simulink model "FW_control"  (R2023b)
settings: Solver=ode45  StartTime=0.0  StopTime=100  RelTol=1e-3
libraries: Fixed_Wing x2
settings Model: Creator=TigerWuu  LastModifiedBy=NCS
settings DebuggingCC: UnconnectedInputMsg=warning  UnconnectedOutputMsg=warning  UnconnectedLineMsg=warning
settings ModelReferenceCC: EnableRefExpFcnMdlSchedulingChecks=on
settings RTWCC: DLArmComputeVersion=19.05

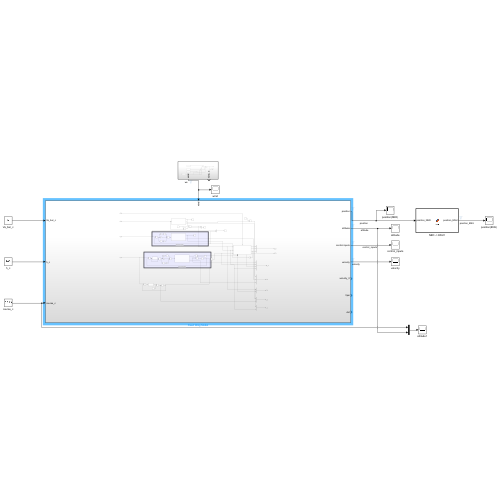
[thumbnail: Simulink's stored preview of the top-level diagram]
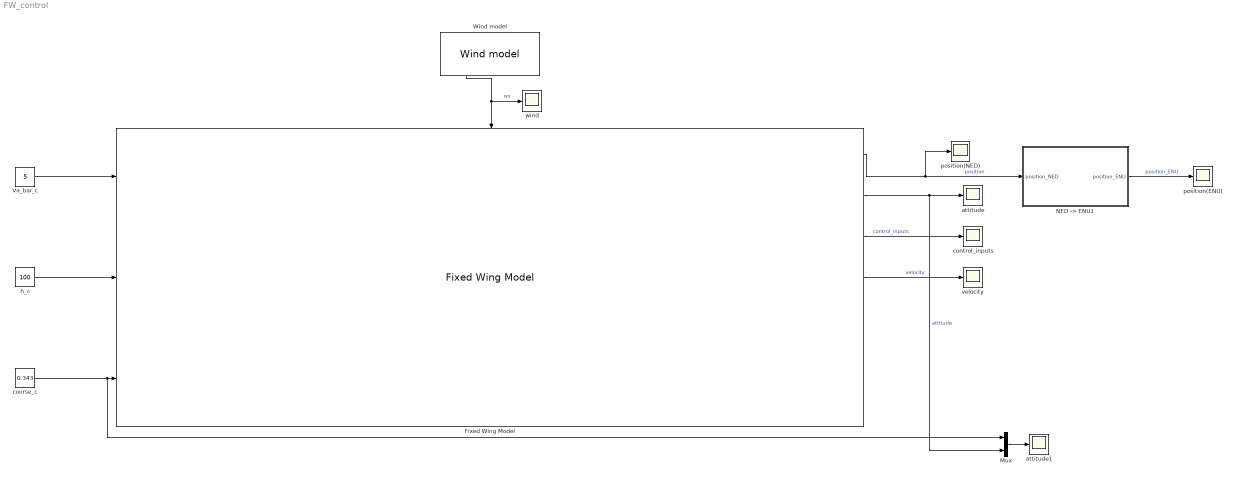
== system FW_control ==
  Fixed Wing Model : Fixed_Wing/Fixed Wing Model  SystemSampleTime=-1  VariantActivationTime=update diagram  AllowFlexibleInterface=on  Latency=0  AutoFrameSizeCalculation=off
      link override Kd_course: Gain=0.1
      link override Ki_course: Gain=0
      link override Kp_course: Gain=1
      settings: SourceProductName=Fixed-Wing Model  PortSchema="{\"entries\":[{\"content\":{\"sides\":[{\"content\":{\"connectorIds\":[\"In1\",\"In2\",\"In3\"]},\"type\":\"ConnectorPlacement.EquallySpacedRectSide\",\"uuid\":\"491080cc-ba33-4dca-9b37-922a1b131a7c\"},{\"content\":{\"connectorIds\":[\"Out1\",\"Out2\",\"Out3\",\"Out4\",\"Out5\",\"Out6\",\"Out7\"],\"side\":\"RIGHT\"},\"type\":\"ConnectorPlacement.EquallySpacedRectSide\",\"uuid\":\"e4e8ca81-264a-41b3-9d62-a2cb565f7b79\"},{\"content\":{\"connectorIds\":[\"In4\"],\"side\":\"TOP\"},\"type\":\"ConnectorPlacement.EquallySpacedRectSide\",\"uuid\":\"52444ebc-de17-4d3c-95e2-2270054ae63e\"}]},\"type\":\"ConnectorPlacement.EquallySpacedConnector\",\"uuid\":\"020d1068-73e8-421c-b651-66bcdf43a07b\"}],\"packageUris\":[\"http://schema.mathworks.com/mf0/Connector/R2020b\"],\"version\":\"1.0\"}"
  Mux : Mux  Inputs=2
  "NED -> ENU1" : MATLAB Function  TreatAsAtomicUnit=on
  Va_bar_c : Constant  Value=5
  Wind model : Fixed_Wing/Wind model  SystemSampleTime=-1  VariantActivationTime=update diagram  AllowFlexibleInterface=on  Latency=0  AutoFrameSizeCalculation=off
      settings: SourceProductName=Fixed-Wing Model  PortSchema="{\"entries\":[{\"content\":{\"sides\":[{\"content\":{},\"type\":\"ConnectorPlacement.EquallySpacedRectSide\",\"uuid\":\"19ef0eb7-c626-45ec-b76b-8668fc024824\"},{\"content\":{\"side\":\"RIGHT\"},\"type\":\"ConnectorPlacement.EquallySpacedRectSide\",\"uuid\":\"89e72569-ab94-4162-a6e2-b425ef08f724\"},{\"content\":{\"side\":\"TOP\"},\"type\":\"ConnectorPlacement.EquallySpacedRectSide\",\"uuid\":\"6d9409e9-6822-4cd9-902f-e5665cb68433\"},{\"content\":{\"connectorIds\":[\"Out1\",\"Out2\"],\"side\":\"BOTTOM\"},\"type\":\"ConnectorPlacement.EquallySpacedRectSide\",\"uuid\":\"39a83352-0924-44fa-be5d-94a7c28bbbf3\"}]},\"type\":\"ConnectorPlacement.EquallySpacedConnector\",\"uuid\":\"6cf6ae00-ef23-42a2-99b2-ca60e191fb03\"}],\"packageUris\":[\"http://schema.mathworks.com/mf0/Connector/R2020b\"],\"version\":\"1.0\"}"
  attitude : Scope
  attitude1 : Scope
  control_inputs : Scope
  course_c : Constant  Value=0.343
  h_c : Constant  Value=100
  position(ENU) : Scope
  position(NED) : Scope
  velocity : Scope
  wind : Scope
  wires:
  Fixed Wing Model/2 -> Mux/2, attitude/1  "attitude"
  Fixed Wing Model/3 -> control_inputs/1  "control_inputs"
  Fixed Wing Model/1 -> position(NED)/1, "NED -> ENU1"/1(position_NED)  "position"
  "NED -> ENU1"/1(position_ENU) -> position(ENU)/1  "position_ENU"
  Wind model/1 -> Fixed Wing Model/4, wind/1  "ws"
  course_c/1 -> Mux/1, Fixed Wing Model/3
  h_c/1 -> Fixed Wing Model/2
  Va_bar_c/1 -> Fixed Wing Model/1
  Fixed Wing Model/4 -> velocity/1  "velocity"
  Mux/1 -> attitude1/1

== matlab function FW_control/NED -> ENU1 ==
  data: position_NED input; position_ENU output
function position_ENU = fcn(position_NED)
R_NED_ENU = [0 1 0;
             1 0 0;
             0 0 -1;];
position_ENU = R_NED_ENU* position_NED;
end
